simulink model "naif"  (R2026a)
settings: Solver=VariableStepAuto  StopTime=t(end)
InitFcn:
  | wtModelFile = get_param(bdroot, 'FileName'); wtProjectRoot = fileparts(fileparts(wtModelFile)); wtScriptsDir = fullfile(wtProjectRoot, 'scripts'); addpath(wtScriptsDir); init_wt(get_wind_case(), false);
model workspace (MAT data in the model file):
  Nrl5mw = Simulink.LookupTable
  Nrl5mw.Table = Simulink.lookuptable.Table
  Nrl5mw.Table.Value = [0.00324958464317  0.00324958464317  0.00342871182387  0.00378195750907  0.00430145700442  0.00497648959739  0.00581708483409  0.0067366262647  0.00771491871349  0.00869835701078  0.00959992599299; 0.0118437200857  0.0118437200857  0.0127087658286  0.014540982327  0.0174679621542  0.022394595811  0.0294771895759  0.0383707887413  0.0478418075681  0.0559163753636  0.0561728348333; 0.0599580773919  0.0599580773919  0.0640834762089  0.0721555686528  0.0839231058338  0.0984682769002  0.112036134022  0.117999874438  0.112412662939  0.0928881826394  0.0412333618321; 0.162160643769  0.162160643769  0.167995847999  0.178881907492  0.192519410401  0.201005075906  0.198824139383  0.17431643879  0.12058472531  0.0381480939525  -0.075485770269; 0.282877500639  0.282877500639  0.289025899865  0.297592205181  0.304695104116  0.289320972066  0.243700713595  0.168131154644  0.0599315282068  -0.0941905168605  -0.285910570062; 0.398893468915  0.398893468915  0.398791838867  0.390546666449  0.371048991486  0.32850296331  0.243876353091  0.116797394354  -0.0625373247481  -0.303237250084  -0.585296699342; 0.450851489569  0.450851489569  0.447832100446  0.436519755531  0.403150980937  0.336582972649  0.212254773161  0.0245263421277  -0.252001751809  -0.600967402132  -0.974327879094; 0.464345202819  0.464345202819  0.46281348753  0.452638435162  0.411696027781  0.326588561618  0.154463569125  -0.113811402208  -0.500304545178  -0.931893902987  -1.46757393977; 0.447551157014  0.447551157014  0.456706312199  0.45081344656  0.407438232487  0.301852716213  0.0710968571135  -0.293763962444  -0.697129499811  -1.21338939823  -2.11658547641; 0.413488526181  0.413488526181  0.425552679088  0.431513081992  0.392237940569  0.2624344305  -0.0459246239423  -0.527464487014  -1.0690672307  -1.82349915742  -2.93809835483; 0.325666749873  0.325666749873  0.376740777889  0.408850107246  0.366134617654  0.206912795208  -0.194305521983  -0.563097565822  -1.24178173936  -2.38510102986  -3.96022300877]
  Nrl5mw.Table.Dimensions = [11 11]
  Nrl5mw.Table.DataType = 'auto'
  Nrl5mw.Table.FieldName = 'Table_Cp'
  Nrl5mw.Breakpoints(1) = Simulink.lookuptable.Breakpoint
  Nrl5mw.Breakpoints(1).Value = [0.5 1.45 2.4 3.35 4.3 5.25 6.2 7.15 8.1 9.05 10]
  Nrl5mw.Breakpoints(1).TunableSizeName = 'N1'
  Nrl5mw.Breakpoints(1).TunableSizeValue = -1
  Nrl5mw.Breakpoints(1).Dimensions = [1 11]
  Nrl5mw.Breakpoints(1).DataType = 'auto'
  Nrl5mw.Breakpoints(1).FieldName = 'BP1_Lambda'
  Nrl5mw.Breakpoints(2) = Simulink.lookuptable.Breakpoint
  Nrl5mw.Breakpoints(2).Value = [0 0.8 1.6 2.4 3.2 4 4.8 5.6 6.4 7.2 8]
  Nrl5mw.Breakpoints(2).TunableSizeName = 'N2'
  Nrl5mw.Breakpoints(2).TunableSizeValue = -1
  Nrl5mw.Breakpoints(2).Dimensions = [1 11]
  Nrl5mw.Breakpoints(2).DataType = 'auto'
  Nrl5mw.Breakpoints(2).FieldName = 'BP2_theta_p'
  Nrl5mw.AllowMultipleInstancesOfTypeToHaveDifferentTableBreakpointSizes = 0
  Nrl5mw.SupportTunableSize = 0
  Nrl5mw.StructTypeInfo = Simulink.lookuptable.StructTypeInfo
  Nrl5mw.StructTypeInfo.Name = 'surfaceBlockParameters_type'
  Nrl5mw.StructTypeInfo.DataScope = 'Auto'
  surfaceBlockParameters = Simulink.LookupTable
  surfaceBlockParameters.Table = Simulink.lookuptable.Table
  surfaceBlockParameters.Table.Value = [0.000629396007942 0.006627327118 0.0623376026933 0.200719842793 0.356874891063 0.394066762825 0.350958924947 0.335467287882 0.311487736698 0.227563659042 0.0973704524374 0.0013612480249 ... (121 elements, 11x11)]
  surfaceBlockParameters.Table.Dimensions = [11 11]
  surfaceBlockParameters.Table.DataType = 'auto'
  surfaceBlockParameters.Table.FieldName = 'Table_Cp_'
  surfaceBlockParameters.Breakpoints(1) = Simulink.lookuptable.Breakpoint
  surfaceBlockParameters.Breakpoints(1).Value = [0.54 2.14 3.74 5.34 6.94 8.54 10.14 11.74 13.34 14.94 16.54]
  surfaceBlockParameters.Breakpoints(1).TunableSizeName = 'N1'
  surfaceBlockParameters.Breakpoints(1).TunableSizeValue = -1
  surfaceBlockParameters.Breakpoints(1).Dimensions = [1 11]
  surfaceBlockParameters.Breakpoints(1).DataType = 'auto'
  surfaceBlockParameters.Breakpoints(1).FieldName = 'BP1_Lambda'
  surfaceBlockParameters.Breakpoints(2) = Simulink.lookuptable.Breakpoint
  surfaceBlockParameters.Breakpoints(2).Value = [-8 -3.7 0.6 4.9 9.2 13.5 17.8 22.1 26.4 30.7 35]
  surfaceBlockParameters.Breakpoints(2).TunableSizeName = 'N2'
  surfaceBlockParameters.Breakpoints(2).TunableSizeValue = -1
  surfaceBlockParameters.Breakpoints(2).Dimensions = [1 11]
  surfaceBlockParameters.Breakpoints(2).DataType = 'auto'
  surfaceBlockParameters.Breakpoints(2).FieldName = 'BP2_Beta'
  surfaceBlockParameters.AllowMultipleInstancesOfTypeToHaveDifferentTableBreakpointSizes = 0
  surfaceBlockParameters.SupportTunableSize = 0
  surfaceBlockParameters.StructTypeInfo = Simulink.lookuptable.StructTypeInfo
  surfaceBlockParameters.StructTypeInfo.Name = 'surfaceBlockParameters_type'
  surfaceBlockParameters.StructTypeInfo.DataScope = 'Auto'
undefined symbols (not defined in the file): Beta_ott, C_rated, GBEff, GBRatio, GenEff, Jeq, Kreg2, Omega_0, Omega_ott_high, Omega_ott_low, R, rho
settings Model: Creator=39388  LastModifiedBy=notes

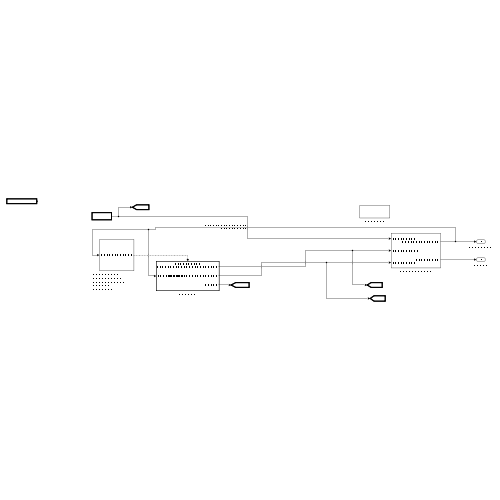
[thumbnail: Simulink's stored preview of the top-level diagram]
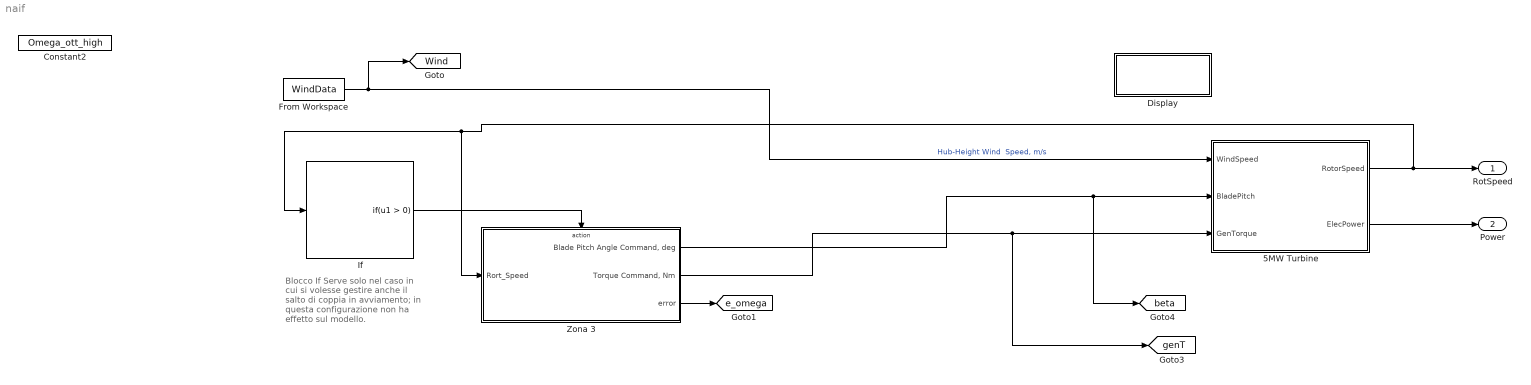
== system naif ==
  note: Blocco If
      | Serve solo nel caso in cui si volesse gestire anche il salto di coppia in avviamento; in questa configurazione non ha effetto sul modello.
  5MW Turbine : Subsystem
  Constant2 : Constant  Value=Omega_ott_high
  Display : Subsystem
  From Workspace : FromWorkspace  VariableName=WindData
  If : If  ShowElse=off  ZeroCross=off
  Zona 3 : Subsystem  TreatAsAtomicUnit=on
  RotSpeed : Outport
  Power : Outport  Port=2
  tag scope: Wind=global, beta=global, e_omega=global, genT=global
  wires:
  If/1 -> Zona 3/Action
  5MW Turbine/2(ElecPower) -> Power/1
  Zona 3/2("Torque Command, Nm") -> [genT], 5MW Turbine/3(GenTorque)
  Zona 3/1("Blade Pitch Angle Command, deg") -> [beta], 5MW Turbine/2(BladePitch)
  From Workspace/1 -> [Wind], 5MW Turbine/1(WindSpeed)  "Hub-Height Wind  Speed, m/s"
  5MW Turbine/1("RotorSpeed ") -> Zona 3/1(Rort_Speed), If/1, RotSpeed/1
  Zona 3/3(error) -> [e_omega]

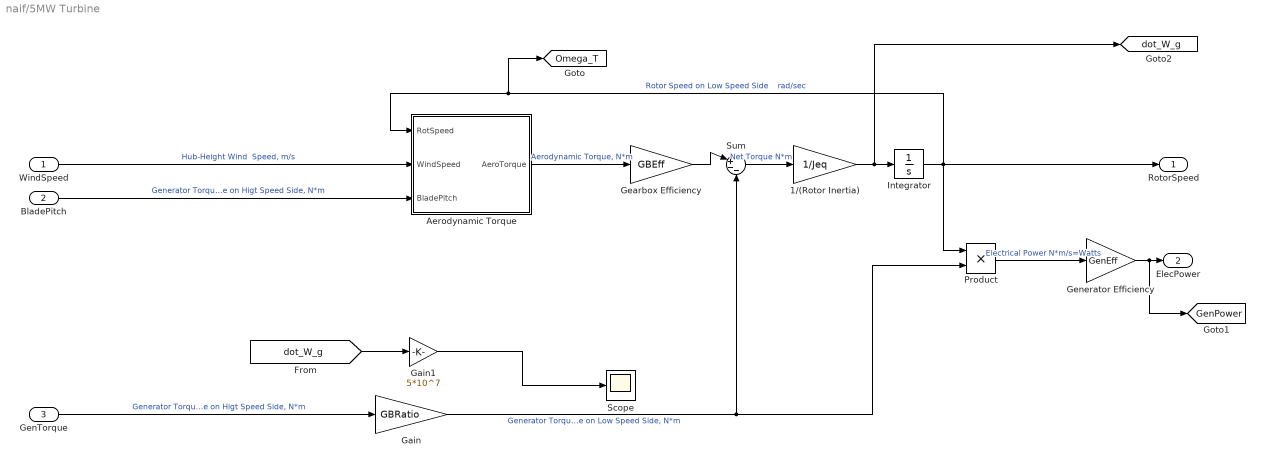
== system naif/5MW Turbine ==
  WindSpeed : Inport
  BladePitch : Inport  Port=2
  GenTorque : Inport  Port=3
  1/(Rotor Inertia) : Gain  Gain=1/Jeq
  Aerodynamic Torque : Subsystem
  Gain : Gain  Gain=GBRatio
  Gain1 : Gain  Gain=5*10^7
  Gearbox Efficiency : Gain  Gain=GBEff
  Generator Efficiency : Gain  Gain=GenEff
  Integrator : Integrator  InitialCondition=Omega_0
  Product : Product  Inputs=**
  Scope : Scope
      settings: ActiveDisplayYMinimum=-1.604705891341E+7  ActiveDisplayYMaximum=3.244093111398E+7
  Sum : Sum  Inputs=|+--
  "RotorSpeed " : Outport
  ElecPower : Outport  Port=2
  tag scope: GenPower=global, Omega_T=global, dot_W_g=global
  wires:
  Integrator/1 -> "RotorSpeed "/1, Product/1, [Omega_T], Aerodynamic Torque/1("RotSpeed ")  "Rotor Speed on Low Speed Side    rad/sec"
  Sum/1 -> 1/(Rotor Inertia)/1  "Net Torque N*m"
  Gearbox Efficiency/1 -> Sum/1
  Gain/1 -> Product/2, Sum/3  "Generator Torque on Low Speed Side, N*m"
  1/(Rotor Inertia)/1 -> [dot_W_g], Integrator/1
  WindSpeed/1 -> Aerodynamic Torque/2(WindSpeed)  "Hub-Height Wind  Speed, m/s"
  Aerodynamic Torque/1(AeroTorque) -> Gearbox Efficiency/1  "Aerodynamic Torque, N*m"
  Product/1 -> Generator Efficiency/1  "Electrical Power N*m/s=Watts"
  Generator Efficiency/1 -> [GenPower], ElecPower/1
  BladePitch/1 -> Aerodynamic Torque/3(BladePitch)  "Generator Torque on Higt Speed Side, N*m"
  GenTorque/1 -> Gain/1  "Generator Torque on Higt Speed Side, N*m"
  [dot_W_g] -> Gain1/1
  Gain1/1 -> Scope/1

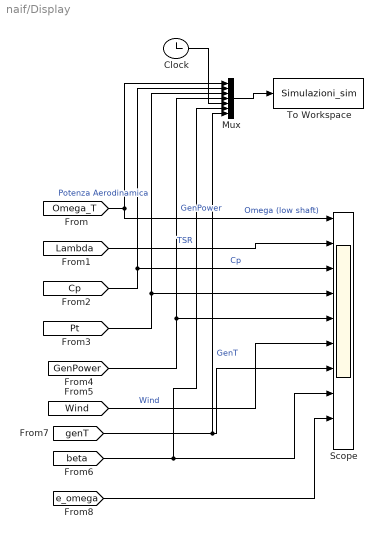
== system naif/Display ==
  Clock : Clock
  Mux : Mux  Inputs=7
  Scope : Scope  NumInputPorts=10
      settings: ActiveDisplayYMinimum=1.01275  ActiveDisplayYMaximum=1.32439
  To Workspace : ToWorkspace  VariableName=Simulazioni_sim  SampleTime=-1
  wires:
  [Omega_T] -> Mux/1, Scope/1  "Omega (low shaft)"
  [Pt] -> Mux/3, Scope/4  "Potenza Aerodinamica"
  [Lambda] -> Scope/2  "TSR"
  [Cp] -> Mux/2, Scope/3  "Cp"
  [GenPower] -> Mux/4, Scope/5  "GenPower"
  [Wind] -> Scope/6  "Wind"
  Mux/1 -> To Workspace/1
  Clock/1 -> Mux/5
  [beta] -> Mux/6, Scope/8
  [genT] -> Mux/7, Scope/7  "GenT"
  [e_omega] -> Scope/9

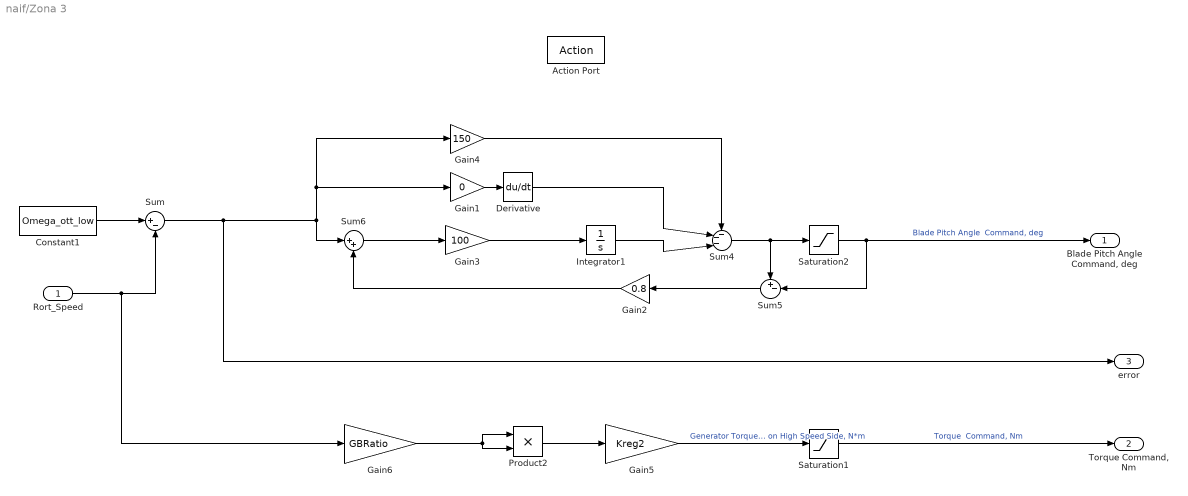
== system naif/Zona 3 ==
  Rort_Speed : Inport
  Action Port : ActionPort  ActionPortLabel=if(u1 > 0)
  Constant1 : Constant  Value=Omega_ott_low
  Derivative : Derivative
  Gain1 : Gain  Gain=0
  Gain2 : Gain  Gain=0.8
  Gain3 : Gain  Gain=100
  Gain4 : Gain  Gain=150
  Gain5 : Gain  Gain=Kreg2
  Gain6 : Gain  Gain=GBRatio
  Integrator1 : Integrator
  Product2 : Product
  Saturation1 : Saturate  UpperLimit=C_rated/GBRatio  LowerLimit=Beta_ott
  Saturation2 : Saturate  UpperLimit=90  LowerLimit=Beta_ott
  Sum : Sum  Inputs=|+-
  Sum4 : Sum  Inputs=---|
  Sum5 : Sum  Inputs=+-|
  Sum6 : Sum  Inputs=|++
  "Blade Pitch Angle Command, deg" : Outport
  "Torque Command, Nm" : Outport  Port=2
  error : Outport  Port=3
  wires:
  Sum4/1 -> Saturation2/1, Sum5/1
  Derivative/1 -> Sum4/2
  Gain4/1 -> Sum4/1
  Sum/1 -> error/1, Sum6/1, Gain4/1, Gain1/1
  Sum5/1 -> Gain2/1
  Sum6/1 -> Gain3/1
  Integrator1/1 -> Sum4/3
  Gain2/1 -> Sum6/2
  Saturation2/1 -> "Blade Pitch Angle Command, deg"/1, Sum5/2  "Blade Pitch Angle  Command, deg"
  Gain3/1 -> Integrator1/1
  Gain1/1 -> Derivative/1
  Constant1/1 -> Sum/1
  Rort_Speed/1 -> Gain6/1, Sum/2
  Gain5/1 -> Saturation1/1  "Generator Torque on High Speed Side, N*m"
  Product2/1 -> Gain5/1
  Gain6/1 -> Product2/2, Product2/1
  Saturation1/1 -> "Torque Command, Nm"/1  "Torque  Command, Nm"

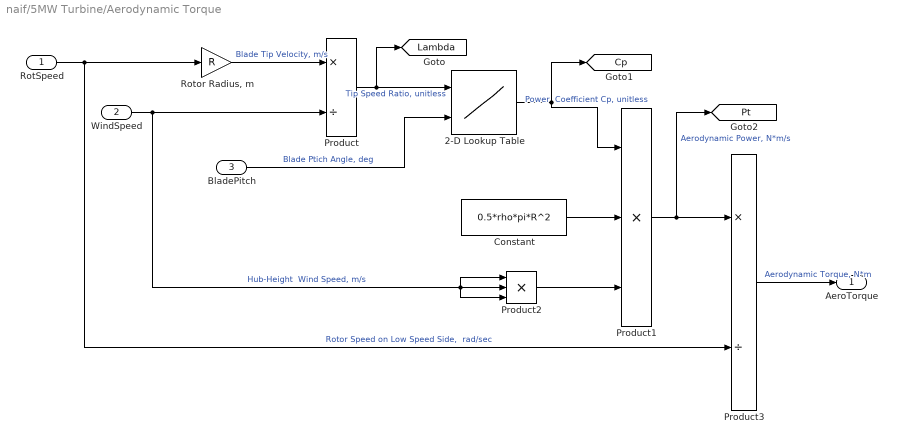
== system naif/5MW Turbine/Aerodynamic Torque ==
  "RotSpeed " : Inport
  WindSpeed : Inport  Port=2
  BladePitch : Inport  Port=3
  2-D Lookup Table : Lookup_n-D  DataSpecification=Lookup table object  LookupTableObject=surfaceBlockParameters  BreakpointsForDimension1=[1:3]  BreakpointsForDimension2=[1:3]  InternalRulePriority=Speed  OutMin=[0]  OutMax=[0.5]  RndMeth=Simplest
      settings: InputPortMap=u0,u1
  Constant : Constant  Value=0.5*rho*pi*R^2
  Product : Product  Inputs=*/
  Product1 : Product  Inputs=***
  Product2 : Product  Inputs=***
  Product3 : Product  Inputs=*/
  "Rotor Radius, m" : Gain  Gain=R
  AeroTorque : Outport
  tag scope: Cp=global, Lambda=global, Pt=global
  wires:
  "RotSpeed "/1 -> Product3/2, "Rotor Radius, m"/1  "Rotor Speed on Low Speed Side,  rad/sec"
  "Rotor Radius, m"/1 -> Product/1  "Blade Tip Velocity, m/s"
  WindSpeed/1 -> Product2/3, Product2/1, Product2/2, Product/2  "Hub-Height  Wind Speed, m/s"
  Product/1 -> 2-D Lookup Table/1, [Lambda]  "Tip Speed Ratio, unitless"
  BladePitch/1 -> 2-D Lookup Table/2  "Blade Ptich Angle, deg"
  2-D Lookup Table/1 -> Product1/1, [Cp]  "Power  Coefficient Cp, unitless"
  Constant/1 -> Product1/2
  Product2/1 -> Product1/3
  Product1/1 -> [Pt], Product3/1  "Aerodynamic Power, N*m/s"
  Product3/1 -> AeroTorque/1  "Aerodynamic Torque, N*m"
